simulink model "simpleModel"  (R2015b)
settings: Solver=FixedStepAuto  StartTime=0.0  StopTime=10.0  RelTol=1e-3
libraries: frdmtfcshieldlib x4, simulink x1
settings Model: ExtModeTrigDuration=5  Creator=dgc14  LastModifiedBy=dgc14
settings OptimizationCC: OptimizeModelRefInitCode=on  LifeSpan=1  MaxStackSize=64
settings HardwareCC: ProdBitPerPointer=32  ProdLargestAtomicInteger=Long  ProdLargestAtomicFloat=Double  ProdWordSize=32  ProdHWDeviceType=ARM Compatible->ARM Cortex
settings RTWCC: SystemTargetFile=ert.tlc  TemplateMakefile=ert_default_tmf  Description=Embedded Coder  Toolchain=GNU Tools for ARM Embedded Processors
settings CodeAppCC: IgnoreCustomStorageClasses=off

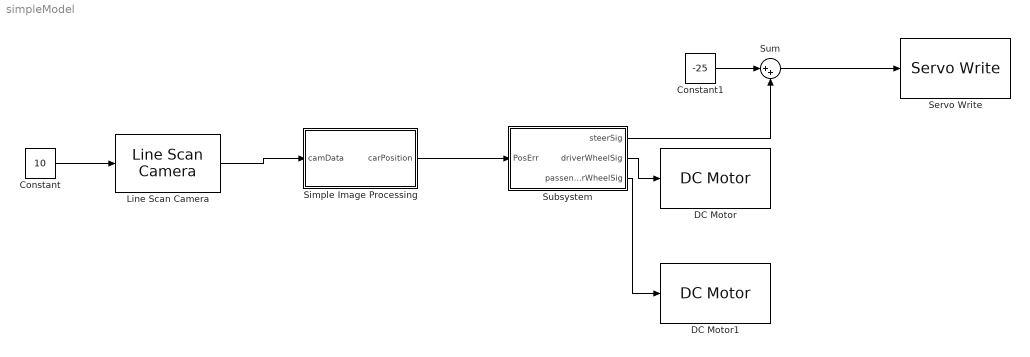
== system simpleModel ==
  Constant : Constant  Value=10  SampleTime=0.1
  Constant1 : Constant  Value=-25
  DC Motor : frdmtfcshieldlib/DC Motor  WhichMotor=A
  DC Motor1 : frdmtfcshieldlib/DC Motor  WhichMotor=B
  Line Scan Camera : frdmtfcshieldlib/Line Scan Camera  CameraHeader=0  SampleTime=0.1
  Servo Write : frdmtfcshieldlib/Servo Write  WhichServo=0  minAngle=-20.0  maxAngle=20.0
  Simple Image Processing : Subsystem
  Subsystem : Subsystem
  Sum : Sum  Inputs=|++
  wires:
  Simple Image Processing/1(carPosition) -> Subsystem/1(PosErr)
  Line Scan Camera/1 -> Simple Image Processing/1(camData)
  Subsystem/2(driverWheelSig) -> DC Motor/1
  Subsystem/3(passengerWheelSig) -> DC Motor1/1
  Constant/1 -> Line Scan Camera/1
  Constant1/1 -> Sum/1
  Subsystem/1(steerSig) -> Sum/2
  Sum/1 -> Servo Write/1

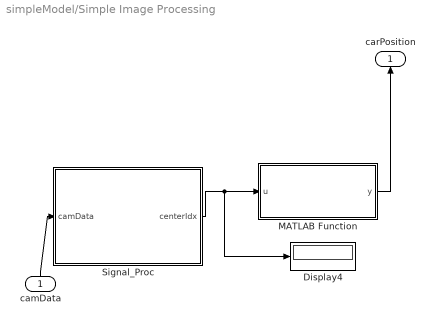
== system simpleModel/Simple Image Processing ==
  camData : Inport
  Display4 : Display
  MATLAB Function : MATLAB Function  TreatAsAtomicUnit=on
  Signal_Proc : MATLAB Function  TreatAsAtomicUnit=on
  carPosition : Outport
  wires:
  Signal_Proc/1(centerIdx) -> Display4/1, MATLAB Function/1(u)
  MATLAB Function/1(y) -> carPosition/1
  camData/1 -> Signal_Proc/1(camData)

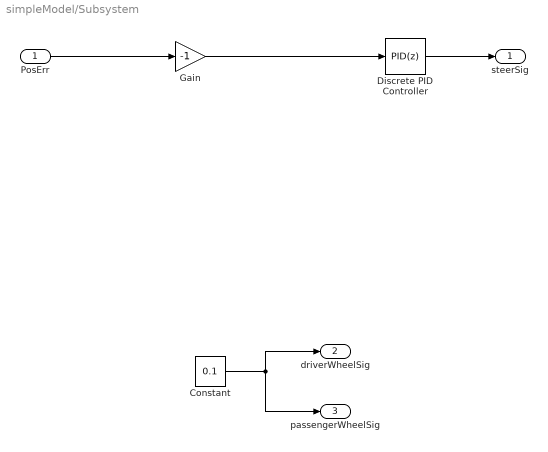
== system simpleModel/Subsystem ==
  PosErr : Inport
  Constant : Constant  Value=0.1
  Discrete PID Controller : simulink/Continuous/PID Controller  Controller=PID  TimeDomain=Discrete-time  SampleTime=0.1  IntegratorMethod=Forward Euler  FilterMethod=Forward Euler  Form=Parallel  UseFilter=on  ControllerParametersSource=internal  P=5  I=3  D=0  N=10  InitialConditionSource=internal  InitialConditionForIntegrator=0  InitialConditionForFilter=0  ExternalReset=none  LimitOutput=on  UpperSaturationLimit=20  LowerSaturationLimit=-20  LinearizeAsGain=off  AntiWindupMode=none  Kb=1  TrackingMode=off  Kt=1  PParamMin=[]  PParamMax=[]  IParamMin=[]  IParamMax=[]  DParamMin=[]  DParamMax=[]  NParamMin=[]  NParamMax=[]  KbParamMin=[]  KbParamMax=[]  KtParamMin=[]  KtParamMax=[]  POutMin=[]  POutMax=[]  IOutMin=[]  IOutMax=[]  DOutMin=[]  DOutMax=[]  NOutMin=[]  NOutMax=[]  KbOutMin=[]  KbOutMax=[]  KtOutMin=[]  KtOutMax=[]  IntegratorOutMin=[]  IntegratorOutMax=[]  FilterOutMin=[]  FilterOutMax=[]  SumOutMin=[]  SumOutMax=[]  SumI1OutMin=[]  SumI1OutMax=[]  SumI2OutMin=[]  SumI2OutMax=[]  SumI3OutMin=[]  SumI3OutMax=[]  SumDOutMin=[]  SumDOutMax=[]  SaturationOutMin=[]  SaturationOutMax=[]  IntegratorContinuousStateAttributes=''  IntegratorStateMustResolveToSignalObject=off  IntegratorRTWStateStorageClass=Auto  FilterContinuousStateAttributes=''  FilterStateMustResolveToSignalObject=off  FilterRTWStateStorageClass=Auto  DifferentiatorICPrevScaledInput=0  DifferentiatorOutMin=[]  DifferentiatorOutMax=[]
  Gain : Gain  Gain=-1
  steerSig : Outport
  driverWheelSig : Outport  Port=2
  passengerWheelSig : Outport  Port=3
  wires:
  Discrete PID Controller/1 -> steerSig/1
  Constant/1 -> passengerWheelSig/1, driverWheelSig/1
  PosErr/1 -> Gain/1
  Gain/1 -> Discrete PID Controller/1

== matlab function simpleModel/Simple Image Processing/MATLAB Function ==
  data: u input; y output
function y = fromIndexToPosition(u)
%#codegen

y = - u + 64;

== matlab function simpleModel/Simple Image Processing/Signal_Proc ==
  data: centerIdx output; camData input
function centerIdx  = centerTrackIdx(camData)

threshold = 5e4;
black = zeros(length(camData),1);
j = 1;
for i=1:length(camData)
    if(camData(i)<threshold)
        black(j)=i;
        j = j+1;
    end
end
j = j-1;
if(j~=0)
    centerIdx = black(floor(j/2));
else
    centerIdx = 64;
end

%%%%%%%%%%%%%%%%%%%%%%%%%%%%%%%%%%%%%%%%%%%%%%%%%%%%%%%%%%%%%%%%%%%%%%%%%%%%%%%%%%%

%find STOP
% 
% h = 29;%camera high
% a = 29.21;%cm (3'-1/2") length from lateral line to center track
% b=60;
% camera_error = 7;
% d = sqrt(b^2+h^2);%diagonal length from camera to view center point
% alfa = atan2(a,d);%optical angle from center to lateral line
% pixel_gap = round(alfa/0.007604262);%pixel from lateral line to center track
% pixel_edge = 64 - pixel_gap + camera_error;%pixel from lateral line to outdoor track
% s1 = 3.81;%cm [1 1/2"] center track to begin stop
% s2 = 13.97;%cm [5 1/2"] center track to end stop
% alfa1 = atan2(s1,d);
% alfa2 = atan2(s2,d);
% s1_pixel = round(alfa1/0.007604262);
% s2_pixel = round(alfa2/0.007604262);
% 
% 
% 
% %         if length(find(camData(64-s2_pixel:64-s1_pixel) < threshold)) > 0.1*(s2_pixel-s1_pixel) &&...
% %             length(find(camData(64+s1_pixel:64+s2_pixel) < threshold)) > 0.1*(s2_pixel-s1_pixel) &&...
% %             length(find(camData(64-s1_pixel:64+s1_pixel) > threshold)) > 0.1*2*s1_pixel
% 
% if length(find(camData(64-s2_pixel-10:64-s1_pixel+10) < threshold)) > 0.6*(s2_pixel-s1_pixel) &&...
%     length(find(camData(64+s1_pixel-10:64+s2_pixel+10) < threshold)) > 0.6*(s2_pixel-s1_pixel) &&...
%     length(find(camData(64-s1_pixel-10:64+s1_pixel+10) > threshold)) > 2*s1_pixel
% 
% %         if length(find(camData(30:98) < threshold)) > (s2_pixel-s1_pixel) &&...
% %             length(find(camData(64-s1_pixel:64+s1_pixel) > threshold)) > 0.1*2*s1_pixel
% 
%     stop = 1;
%     centerIdx=64;
% end
% 
% if length(find(camData(40:60) < threshold)) > 0.55*20 &&...
%     length(find(camData(70:90) < threshold)) > 0.55*20 &&...
%     length(find(camData(60:70) > threshold)) > 0.55*10
% 
% %         if length(find(camData(30:98) < threshold)) > (s2_pixel-s1_pixel) &&...
% %             length(find(camData(64-s1_pixel:64+s1_pixel) > threshold)) > 0.1*2*s1_pixel
% 
%     stop = 1;
%     centerIdx=64;
% end
